simulink model "tunnelSystem"  (R2023b)
settings: Solver=VariableStepAuto  StartTime=0.0  StopTime=10.0  RelTol=1e-3
settings Model: Creator=user  LastModifiedBy=user

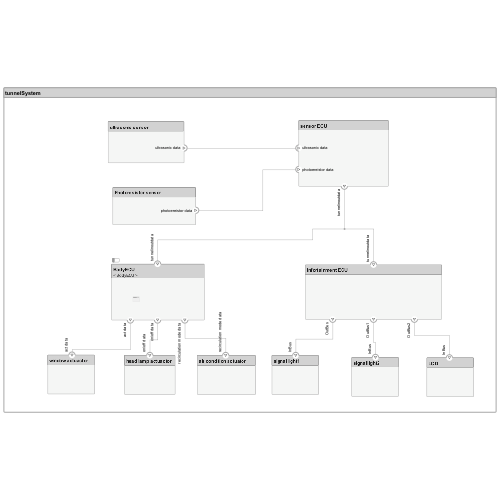
[thumbnail: Simulink's stored preview of the top-level diagram]
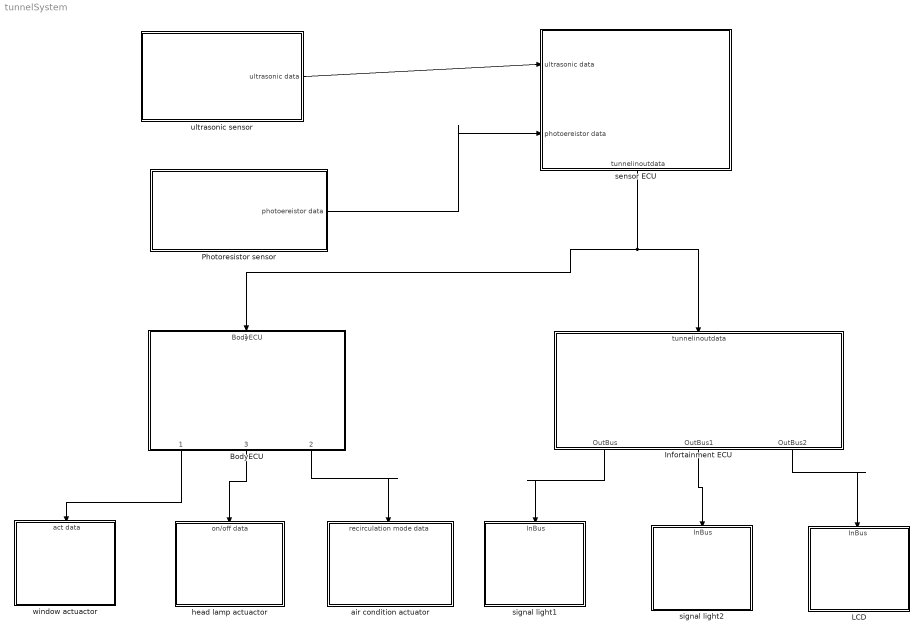
== system tunnelSystem ==
  BodyECU : ModelReference  ModelNameDialog=BodyECU  SimulationMode=Normal  ScheduleRates=on  ScheduleRatesWith=Schedule Editor  ModelReferenceVersion=1.2
      settings: PortSchema="{\"entries\":[{\"content\":{\"headerSize\":38,\"margin\":15,\"minimumSpacing\":25,\"sides\":[{\"content\":{},\"type\":\"ConnectorPlacement.EquallySpacedRectSide\",\"uuid\":\"82d721e7-060c-4f1d-a7c3-17f4aadc223b\"},{\"content\":{\"side\":\"RIGHT\"},\"type\":\"ConnectorPlacement.EquallySpacedRectSide\",\"uuid\":\"73c3a99e-52fc-4b95-9555-7d35ba7fb510\"},{\"content\":{\"connectorIds\":[\"In1\"],\"side\":\"TOP\"},\"type\":\"ConnectorPlacement.EquallySpacedRectSide\",\"uuid\":\"6139ad0a-3299-4ed9-a3a6-8907c5a28ce2\"},{\"content\":{\"connectorIds\":[\"Out1\",\"Out3\",\"Out2\"],\"side\":\"BOTTOM\"},\"type\":\"ConnectorPlacement.EquallySpacedRectSide\",\"uuid\":\"77aed3b8-5be3-4a22-91dc-1424ab859804\"}]},\"type\":\"ConnectorPlacement.EquallySpacedConnector\",\"uuid\":\"27c660f2-6da6-40a4-bd82-ae87fc0ec416\"}],\"packageUris\":[\"http://schema.mathworks.com/mf0/Connector/R2020b\"],\"version\":\"1.0\"}"
  Infortainment ECU : Subsystem
      settings: PortSchema="{\"entries\":[{\"content\":{\"headerSize\":26,\"margin\":15,\"minimumSpacing\":25,\"sides\":[{\"content\":{},\"type\":\"ConnectorPlacement.EquallySpacedRectSide\",\"uuid\":\"82d721e7-060c-4f1d-a7c3-17f4aadc223b\"},{\"content\":{\"side\":\"RIGHT\"},\"type\":\"ConnectorPlacement.EquallySpacedRectSide\",\"uuid\":\"73c3a99e-52fc-4b95-9555-7d35ba7fb510\"},{\"content\":{\"connectorIds\":[\"In1\"],\"side\":\"TOP\"},\"type\":\"ConnectorPlacement.EquallySpacedRectSide\",\"uuid\":\"6139ad0a-3299-4ed9-a3a6-8907c5a28ce2\"},{\"content\":{\"connectorIds\":[\"Out1\",\"Out2\",\"Out3\"],\"side\":\"BOTTOM\"},\"type\":\"ConnectorPlacement.EquallySpacedRectSide\",\"uuid\":\"18e6e969-fc09-4952-b057-314d2ea0972c\"}]},\"type\":\"ConnectorPlacement.EquallySpacedConnector\",\"uuid\":\"27c660f2-6da6-40a4-bd82-ae87fc0ec416\"}],\"packageUris\":[\"http://schema.mathworks.com/mf0/Connector/R2020b\"],\"version\":\"1.0\"}"
  LCD : Subsystem
      settings: PortSchema="{\"entries\":[{\"content\":{\"headerSize\":26,\"margin\":15,\"minimumSpacing\":25,\"sides\":[{\"content\":{},\"type\":\"ConnectorPlacement.EquallySpacedRectSide\",\"uuid\":\"c2694ceb-c454-43a7-a078-9109fe6945fb\"},{\"content\":{\"side\":\"RIGHT\"},\"type\":\"ConnectorPlacement.EquallySpacedRectSide\",\"uuid\":\"7bef276b-d1c8-4a38-addf-eaedef915d80\"},{\"content\":{\"connectorIds\":[\"In1\"],\"side\":\"TOP\"},\"type\":\"ConnectorPlacement.EquallySpacedRectSide\",\"uuid\":\"1bd770ea-f80d-40d8-aca0-93c85bc890e7\"}]},\"type\":\"ConnectorPlacement.EquallySpacedConnector\",\"uuid\":\"fb0d4389-e8c9-4635-a0c4-617996040e89\"}],\"packageUris\":[\"http://schema.mathworks.com/mf0/Connector/R2020b\"],\"version\":\"1.0\"}"
  Photoresistor sensor : Subsystem
      settings: PortSchema="{\"entries\":[{\"content\":{\"headerSize\":26,\"margin\":15,\"minimumSpacing\":25,\"sides\":[{\"content\":{},\"type\":\"ConnectorPlacement.EquallySpacedRectSide\",\"uuid\":\"82d721e7-060c-4f1d-a7c3-17f4aadc223b\"},{\"content\":{\"connectorIds\":[\"Out1\"],\"side\":\"RIGHT\"},\"type\":\"ConnectorPlacement.EquallySpacedRectSide\",\"uuid\":\"73c3a99e-52fc-4b95-9555-7d35ba7fb510\"},{\"content\":{\"side\":\"TOP\"},\"type\":\"ConnectorPlacement.EquallySpacedRectSide\",\"uuid\":\"6139ad0a-3299-4ed9-a3a6-8907c5a28ce2\"},{\"content\":{\"side\":\"BOTTOM\"},\"type\":\"ConnectorPlacement.EquallySpacedRectSide\",\"uuid\":\"8ba6b9d1-dce5-41ee-a39f-c3b482b663b4\"}]},\"type\":\"ConnectorPlacement.EquallySpacedConnector\",\"uuid\":\"27c660f2-6da6-40a4-bd82-ae87fc0ec416\"}],\"packageUris\":[\"http://schema.mathworks.com/mf0/Connector/R2020b\"],\"version\":\"1.0\"}"
  air condition actuator : Subsystem
      settings: PortSchema="{\"entries\":[{\"content\":{\"headerSize\":26,\"margin\":15,\"minimumSpacing\":25,\"sides\":[{\"content\":{},\"type\":\"ConnectorPlacement.EquallySpacedRectSide\",\"uuid\":\"c2694ceb-c454-43a7-a078-9109fe6945fb\"},{\"content\":{\"side\":\"RIGHT\"},\"type\":\"ConnectorPlacement.EquallySpacedRectSide\",\"uuid\":\"7bef276b-d1c8-4a38-addf-eaedef915d80\"},{\"content\":{\"connectorIds\":[\"In1\"],\"side\":\"TOP\"},\"type\":\"ConnectorPlacement.EquallySpacedRectSide\",\"uuid\":\"1bd770ea-f80d-40d8-aca0-93c85bc890e7\"}]},\"type\":\"ConnectorPlacement.EquallySpacedConnector\",\"uuid\":\"fb0d4389-e8c9-4635-a0c4-617996040e89\"}],\"packageUris\":[\"http://schema.mathworks.com/mf0/Connector/R2020b\"],\"version\":\"1.0\"}"
  head lamp actuactor : Subsystem
      settings: PortSchema="{\"entries\":[{\"content\":{\"headerSize\":26,\"margin\":15,\"minimumSpacing\":25,\"sides\":[{\"content\":{},\"type\":\"ConnectorPlacement.EquallySpacedRectSide\",\"uuid\":\"c2694ceb-c454-43a7-a078-9109fe6945fb\"},{\"content\":{\"side\":\"RIGHT\"},\"type\":\"ConnectorPlacement.EquallySpacedRectSide\",\"uuid\":\"7bef276b-d1c8-4a38-addf-eaedef915d80\"},{\"content\":{\"connectorIds\":[\"In1\"],\"side\":\"TOP\"},\"type\":\"ConnectorPlacement.EquallySpacedRectSide\",\"uuid\":\"1bd770ea-f80d-40d8-aca0-93c85bc890e7\"}]},\"type\":\"ConnectorPlacement.EquallySpacedConnector\",\"uuid\":\"fb0d4389-e8c9-4635-a0c4-617996040e89\"}],\"packageUris\":[\"http://schema.mathworks.com/mf0/Connector/R2020b\"],\"version\":\"1.0\"}"
  sensor ECU : Subsystem
      settings: PortSchema="{\"entries\":[{\"content\":{\"headerSize\":26,\"margin\":15,\"minimumSpacing\":25,\"sides\":[{\"content\":{\"connectorIds\":[\"In2\",\"In1\"]},\"type\":\"ConnectorPlacement.EquallySpacedRectSide\",\"uuid\":\"c2694ceb-c454-43a7-a078-9109fe6945fb\"},{\"content\":{\"side\":\"RIGHT\"},\"type\":\"ConnectorPlacement.EquallySpacedRectSide\",\"uuid\":\"7bef276b-d1c8-4a38-addf-eaedef915d80\"},{\"content\":{\"side\":\"TOP\"},\"type\":\"ConnectorPlacement.EquallySpacedRectSide\",\"uuid\":\"1bd770ea-f80d-40d8-aca0-93c85bc890e7\"},{\"content\":{\"connectorIds\":[\"Out1\"],\"side\":\"BOTTOM\"},\"type\":\"ConnectorPlacement.EquallySpacedRectSide\",\"uuid\":\"31934fb4-0c55-4f25-a480-e14738ddd1ed\"}]},\"type\":\"ConnectorPlacement.EquallySpacedConnector\",\"uuid\":\"fb0d4389-e8c9-4635-a0c4-617996040e89\"}],\"packageUris\":[\"http://schema.mathworks.com/mf0/Connector/R2020b\"],\"version\":\"1.0\"}"
  signal light1 : Subsystem
      settings: PortSchema="{\"entries\":[{\"content\":{\"headerSize\":26,\"margin\":15,\"minimumSpacing\":25,\"sides\":[{\"content\":{},\"type\":\"ConnectorPlacement.EquallySpacedRectSide\",\"uuid\":\"c2694ceb-c454-43a7-a078-9109fe6945fb\"},{\"content\":{\"side\":\"RIGHT\"},\"type\":\"ConnectorPlacement.EquallySpacedRectSide\",\"uuid\":\"7bef276b-d1c8-4a38-addf-eaedef915d80\"},{\"content\":{\"connectorIds\":[\"In1\"],\"side\":\"TOP\"},\"type\":\"ConnectorPlacement.EquallySpacedRectSide\",\"uuid\":\"1bd770ea-f80d-40d8-aca0-93c85bc890e7\"}]},\"type\":\"ConnectorPlacement.EquallySpacedConnector\",\"uuid\":\"fb0d4389-e8c9-4635-a0c4-617996040e89\"}],\"packageUris\":[\"http://schema.mathworks.com/mf0/Connector/R2020b\"],\"version\":\"1.0\"}"
  signal light2 : Subsystem
      settings: PortSchema="{\"entries\":[{\"content\":{\"headerSize\":26,\"margin\":15,\"minimumSpacing\":25,\"sides\":[{\"content\":{},\"type\":\"ConnectorPlacement.EquallySpacedRectSide\",\"uuid\":\"c2694ceb-c454-43a7-a078-9109fe6945fb\"},{\"content\":{\"side\":\"RIGHT\"},\"type\":\"ConnectorPlacement.EquallySpacedRectSide\",\"uuid\":\"7bef276b-d1c8-4a38-addf-eaedef915d80\"},{\"content\":{\"connectorIds\":[\"In1\"],\"side\":\"TOP\"},\"type\":\"ConnectorPlacement.EquallySpacedRectSide\",\"uuid\":\"1bd770ea-f80d-40d8-aca0-93c85bc890e7\"}]},\"type\":\"ConnectorPlacement.EquallySpacedConnector\",\"uuid\":\"fb0d4389-e8c9-4635-a0c4-617996040e89\"}],\"packageUris\":[\"http://schema.mathworks.com/mf0/Connector/R2020b\"],\"version\":\"1.0\"}"
  "ultrasonic sensor " : Subsystem
      settings: PortSchema="{\"entries\":[{\"content\":{\"headerSize\":26,\"margin\":15,\"minimumSpacing\":25,\"sides\":[{\"content\":{},\"type\":\"ConnectorPlacement.EquallySpacedRectSide\",\"uuid\":\"82d721e7-060c-4f1d-a7c3-17f4aadc223b\"},{\"content\":{\"connectorIds\":[\"Out1\"],\"side\":\"RIGHT\"},\"type\":\"ConnectorPlacement.EquallySpacedRectSide\",\"uuid\":\"73c3a99e-52fc-4b95-9555-7d35ba7fb510\"},{\"content\":{\"side\":\"TOP\"},\"type\":\"ConnectorPlacement.EquallySpacedRectSide\",\"uuid\":\"6139ad0a-3299-4ed9-a3a6-8907c5a28ce2\"}]},\"type\":\"ConnectorPlacement.EquallySpacedConnector\",\"uuid\":\"27c660f2-6da6-40a4-bd82-ae87fc0ec416\"}],\"packageUris\":[\"http://schema.mathworks.com/mf0/Connector/R2020b\"],\"version\":\"1.0\"}"
  window actuactor : Subsystem
      settings: PortSchema="{\"entries\":[{\"content\":{\"headerSize\":26,\"margin\":15,\"minimumSpacing\":25,\"sides\":[{\"content\":{},\"type\":\"ConnectorPlacement.EquallySpacedRectSide\",\"uuid\":\"c2694ceb-c454-43a7-a078-9109fe6945fb\"},{\"content\":{\"side\":\"RIGHT\"},\"type\":\"ConnectorPlacement.EquallySpacedRectSide\",\"uuid\":\"7bef276b-d1c8-4a38-addf-eaedef915d80\"},{\"content\":{\"connectorIds\":[\"In1\"],\"side\":\"TOP\"},\"type\":\"ConnectorPlacement.EquallySpacedRectSide\",\"uuid\":\"1bd770ea-f80d-40d8-aca0-93c85bc890e7\"}]},\"type\":\"ConnectorPlacement.EquallySpacedConnector\",\"uuid\":\"fb0d4389-e8c9-4635-a0c4-617996040e89\"}],\"packageUris\":[\"http://schema.mathworks.com/mf0/Connector/R2020b\"],\"version\":\"1.0\"}"
  wires:
  "ultrasonic sensor "/1(ultrasonic data) -> sensor ECU/2(ultrasonic data)
  Photoresistor sensor/1(photoereistor data) -> sensor ECU/1(photoereistor data)
  Infortainment ECU/1(OutBus) -> signal light1/1(InBus)
  Infortainment ECU/2(OutBus1) -> signal light2/1(InBus)
  Infortainment ECU/3(OutBus2) -> LCD/1(InBus)
  sensor ECU/1(tunnelinoutdata) -> BodyECU/1, Infortainment ECU/1(tunnelinoutdata)
  BodyECU/1 -> window actuactor/1(act data)
  BodyECU/3 -> head lamp actuactor/1(on/off data)
  BodyECU/2 -> air condition actuator/1(recirculation mode data)

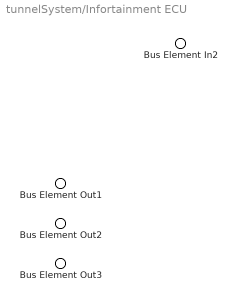
== system tunnelSystem/Infortainment ECU ==
  Bus Element In2 : Inport  PortName=tunnelinoutdata
  Bus Element Out1 : Outport  PortName=OutBus
  Bus Element Out2 : Outport  Port=2  PortName=OutBus1
  Bus Element Out3 : Outport  Port=3  PortName=OutBus2

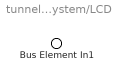
== system tunnelSystem/LCD ==
  Bus Element In1 : Inport  PortName=InBus

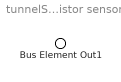
== system tunnelSystem/Photoresistor sensor ==
  Bus Element Out1 : Outport  PortName=photoereistor data

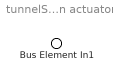
== system tunnelSystem/air condition actuator ==
  Bus Element In1 : Inport  PortName=recirculation mode data

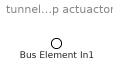
== system tunnelSystem/head lamp actuactor ==
  Bus Element In1 : Inport  PortName=on/off data

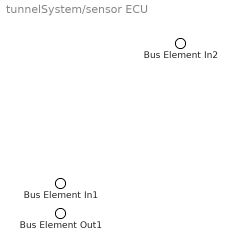
== system tunnelSystem/sensor ECU ==
  Bus Element In2 : Inport  PortName=photoereistor data
  Bus Element In1 : Inport  Port=2  PortName=ultrasonic data
  Bus Element Out1 : Outport  PortName=tunnelinoutdata

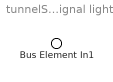
== system tunnelSystem/signal light1 ==
  Bus Element In1 : Inport  PortName=InBus

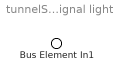
== system tunnelSystem/signal light2 ==
  Bus Element In1 : Inport  PortName=InBus

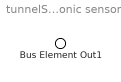
== system tunnelSystem/ultrasonic sensor  ==
  Bus Element Out1 : Outport  PortName=ultrasonic data

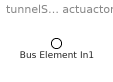
== system tunnelSystem/window actuactor ==
  Bus Element In1 : Inport  PortName=act data
